simulink library "plant"  (R2020a)
settings: Solver=VariableStepAuto  StartTime=0.0  StopTime=10.0  RelTol=1e-3
undefined symbols (not defined in the file): aeroCent, AoA, AoA_vals, CD_vals, CL_vals, gravAccl, init_azim, init_azimRate, init_elev, init_elevRate, init_R, kiteMass, refArea, rho
libraries: threeDofDynamics x1, calculate_vector_magnitude x1, calc_B_FandMaero x1, calc_G_Fgrav x1, rotationFromGroundToTangent x1
settings Model: Creator=Ayaz  LastModifiedBy=Ayaz

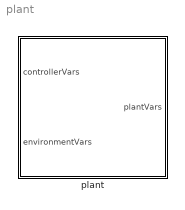
== system plant ==
  plant : Subsystem  mask{AoA=AoA, init_radius=init_R, init_azim=init_azim, init_elev=init_elev, init_dAzim=init_azimRate, init_dElev=init_elevRate, gravEnable=on, fluidEnable=on, mass=kiteMass, refArea=refArea, aeroCent=aeroCent, AoA_vals=AoA_vals, CL_vals=CL_vals, CD_vals=CD_vals, flowDensity=rho, gravAccel=gravAccl}
      mask prompts: AoA "Angle of attack [deg]"; init_radius "Initial sphere radius [m]"; init_azim "Initial azimuth angle [rad]"; init_elev "Initial elevation angle [rad]"; init_dAzim "Initial azimuth angle rate [rad/s]"; init_dElev "Initial elevation angle rate [rad/s]"; gravEnable "Gravity loads enabled?"; fluidEnable "Fluid loads enabled?"; mass "Kite mass [kg]"; refArea "Reference area [m^2]"; aeroCent "Aerodynamic center [m]"; AoA_vals "Angle of attack values [deg]"; CL_vals "Lift coeffcient values [-]"; CD_vals "Drag coefficient values [-]"; flowDensity "Flow density [kg/m^3]"; gravAccel "Gravitational acceleration [m/s^2]"
      mask TypeOptions init_radius: 3 DOF dynamics/init_radius
      mask TypeOptions init_azim: 3 DOF dynamics/init_azim
      mask TypeOptions init_elev: 3 DOF dynamics/init_elev
      mask TypeOptions init_dAzim: 3 DOF dynamics/init_dAzim
      mask TypeOptions init_dElev: 3 DOF dynamics/init_dElev
      mask TypeOptions mass: 3 DOF dynamics/mass | gravForce/mass
      mask TypeOptions refArea: fluidLoads/refArea
      mask TypeOptions aeroCent: fluidLoads/aeroCent
      mask TypeOptions AoA_vals: fluidLoads/AoA_vals
      mask TypeOptions CL_vals: fluidLoads/CL_vals
      mask TypeOptions CD_vals: fluidLoads/CD_vals
      mask TypeOptions flowDensity: fluidLoads/flowDensity
      mask TypeOptions gravAccel: gravForce/gravAccel
      mask DialogControl ParameterGroupVar Prompt: Simulation parameters
      mask DialogControl Container3 Prompt: Kite parameters
      mask DialogControl Container4 Prompt: Environment

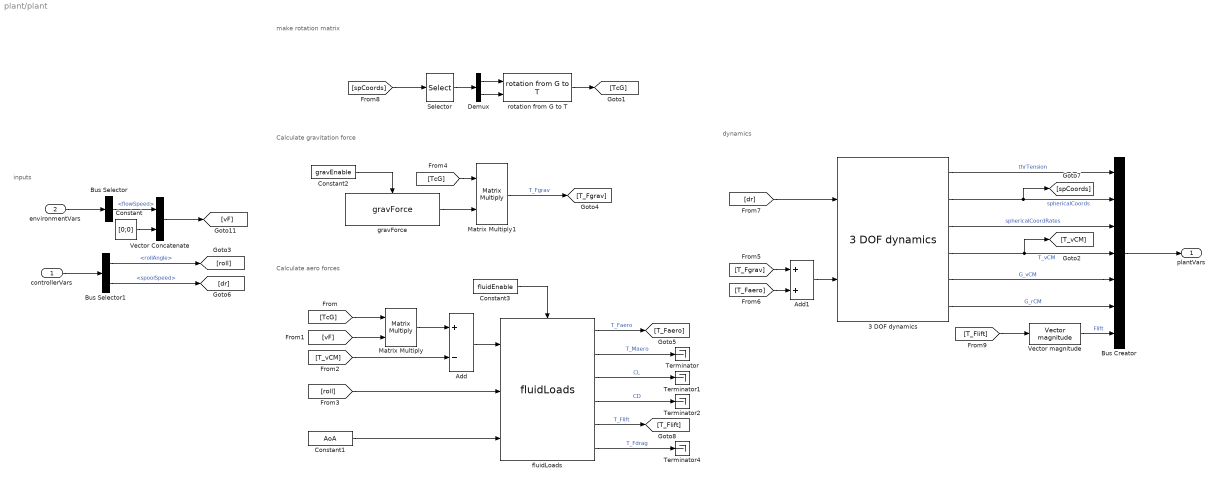
== system plant/plant ==
  note: dynamics
  note: make rotation matrix
  note: inputs
  note: Calculate gravitation force
  note: Calculate aero forces
  controllerVars : Inport
  environmentVars : Inport  Port=2
  3 DOF dynamics : threeDofDynamics/3 DOF dynamics  mass=mass  init_radius=init_radius  init_azim=init_azim  init_elev=init_elev  init_dAzim=init_dAzim  init_dElev=init_dElev
  Add : Sum  Inputs=+-
  Add1 : Sum
  Bus Creator : BusCreator  Inputs=7
  Bus Selector : BusSelector  OutputSignals=flowSpeed
  Bus Selector1 : BusSelector  OutputSignals=rollAngle,spoolSpeed
  Constant : Constant  Value=[0;0]  VectorParams1D=off
  Constant1 : Constant  Value=AoA  VectorParams1D=off
  Constant2 : Constant  Value=gravEnable  VectorParams1D=off  OutDataTypeStr=boolean
  Constant3 : Constant  Value=fluidEnable  VectorParams1D=off  OutDataTypeStr=boolean
  Demux : Demux  Outputs=2
  Matrix Multiply : Product  Multiplication=Matrix(*)
  Matrix Multiply1 : Product  Multiplication=Matrix(*)
  Selector : Selector  InputPortWidth=3  IndexOptions=Index vector (dialog)  Indices=[1 2]  OutputSizes=1
  Terminator{,1..2,4} (4 alike) : Terminator
  Vector Concatenate : Concatenate
  Vector magnitude : calculate_vector_magnitude/Vector magnitude  SystemSampleTime=-1  Latency=0  AutoFrameSizeCalculation=off
  fluidLoads : calc_B_FandMaero/fluidLoads  refArea=refArea  aeroCent=aeroCent  flowDensity=flowDensity  AoA_vals=AoA_vals  CL_vals=CL_vals  CD_vals=CD_vals
  gravForce : calc_G_Fgrav/gravForce  mass=mass  gravAccel=gravAccel
  rotation from G to T : rotationFromGroundToTangent/rotation from G to T  SystemSampleTime=-1  Latency=0  AutoFrameSizeCalculation=off
  plantVars : Outport
  wires:
  Bus Creator/1 -> plantVars/1
  3 DOF dynamics/1 -> Bus Creator/1  "thrTension"
  environmentVars/1 -> Bus Selector/1
  Bus Selector/1 -> Vector Concatenate/1  "<flowSpeed>"
  Constant/1 -> Vector Concatenate/2
  Vector Concatenate/1 -> [vF]
  [TcG] -> Matrix Multiply/1
  [vF] -> Matrix Multiply/2
  3 DOF dynamics/4 -> Bus Creator/4, [T_vCM]  "T_vCM"
  Matrix Multiply/1 -> Add/1
  [T_vCM] -> Add/2
  Add/1 -> fluidLoads/1
  Bus Selector1/1 -> [roll]  "<rollAngle>"
  [roll] -> fluidLoads/2
  Constant1/1 -> fluidLoads/3
  [TcG] -> Matrix Multiply1/1
  gravForce/1 -> Matrix Multiply1/2
  Add1/1 -> 3 DOF dynamics/2
  Matrix Multiply1/1 -> [T_Fgrav]  "T_Fgrav"
  fluidLoads/1 -> [T_Faero]  "T_Faero"
  fluidLoads/2 -> Terminator/1  "T_Maero"
  fluidLoads/3 -> Terminator1/1  "CL"
  fluidLoads/5 -> [T_Flift]  "T_Flift"
  fluidLoads/4 -> Terminator2/1  "CD"
  fluidLoads/6 -> Terminator4/1  "T_Fdrag"
  [T_Fgrav] -> Add1/1
  [T_Faero] -> Add1/2
  Bus Selector1/2 -> [dr]  "<spoolSpeed>"
  [dr] -> 3 DOF dynamics/1
  controllerVars/1 -> Bus Selector1/1
  rotation from G to T/1 -> [TcG]
  Demux/1 -> rotation from G to T/1
  Selector/1 -> Demux/1
  Demux/2 -> rotation from G to T/2
  [spCoords] -> Selector/1
  3 DOF dynamics/2 -> Bus Creator/2, [spCoords]  "sphericalCoords"
  3 DOF dynamics/3 -> Bus Creator/3  "sphericalCoordRates"
  3 DOF dynamics/5 -> Bus Creator/5  "G_vCM"
  3 DOF dynamics/6 -> Bus Creator/6  "G_rCM"
  Constant2/1 -> gravForce/Enable
  Constant3/1 -> fluidLoads/Enable
  Vector magnitude/1 -> Bus Creator/7  "Flift"
  [T_Flift] -> Vector magnitude/1
